simulink model "torque_controller"  (R2019a)
settings: Solver=VariableStepAuto  StartTime=0.0  StopTime=10.0  RelTol=1e-3
undefined symbols (not defined in the file): Kd, Ki, Kp
libraries: simulink x3
settings Model: Creator=Greg  LastModifiedBy=erino

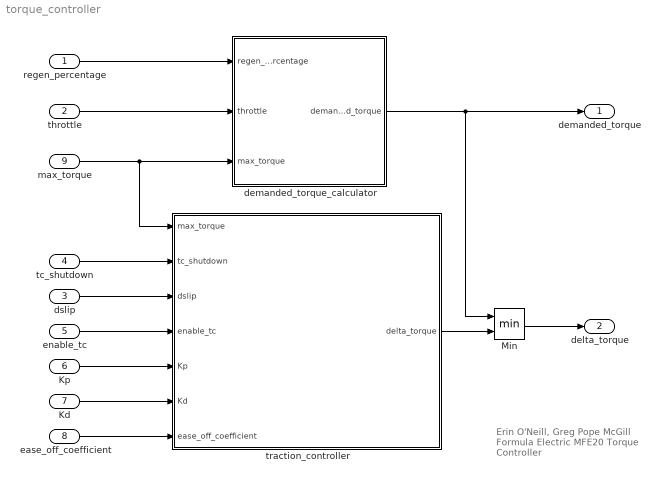
== system torque_controller ==
  note: Erin O'Neill, Greg Pope
      | McGill Formula Electric
      |
      | MFE20 Torque
      | Controller
  regen_percentage : Inport
  throttle : Inport  Port=2
  dslip : Inport  Port=3
  tc_shutdown : Inport  Port=4
  enable_tc : Inport  Port=5
  Kp : Inport  Port=6
  Kd : Inport  Port=7
  ease_off_coefficient : Inport  Port=8
  max_torque : Inport  Port=9
  Min : MinMax  Inputs=2
  demanded_torque_calculator : Subsystem
  traction_controller : Subsystem
  demanded_torque : Outport
  delta_torque : Outport  Port=2
  wires:
  Kp/1 -> traction_controller/5(Kp)
  regen_percentage/1 -> demanded_torque_calculator/1(regen_percentage)
  enable_tc/1 -> traction_controller/4(enable_tc)
  Min/1 -> delta_torque/1
  Kd/1 -> traction_controller/6(Kd)
  ease_off_coefficient/1 -> traction_controller/7(ease_off_coefficient)
  tc_shutdown/1 -> traction_controller/2(tc_shutdown)
  demanded_torque_calculator/1(demanded_torque) -> demanded_torque/1, Min/1
  dslip/1 -> traction_controller/3(dslip)
  traction_controller/1(delta_torque) -> Min/2
  throttle/1 -> demanded_torque_calculator/2(throttle)
  max_torque/1 -> traction_controller/1(max_torque), demanded_torque_calculator/3(max_torque)

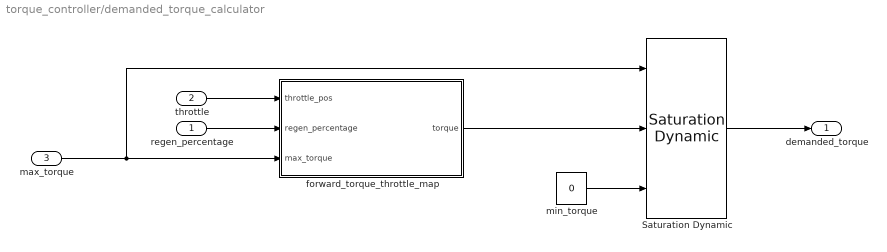
== system torque_controller/demanded_torque_calculator ==
  regen_percentage : Inport
  throttle : Inport  Port=2
  max_torque : Inport  Port=3
  Saturation Dynamic : simulink/Discontinuities/Saturation Dynamic  OutMin=[]  OutMax=[]  OutDataTypeStr=Inherit: Same as second input  OutDataType=fixdt(1, 16)  OutScaling=2^-10  DoSatur=off
  forward_torque_throttle_map : MATLAB Function  TreatAsAtomicUnit=on
  min_torque : Constant  Value=0
  demanded_torque : Outport
  wires:
  max_torque/1 -> Saturation Dynamic/1, forward_torque_throttle_map/3(max_torque)
  forward_torque_throttle_map/1(torque) -> Saturation Dynamic/2
  Saturation Dynamic/1 -> demanded_torque/1
  throttle/1 -> forward_torque_throttle_map/1(throttle_pos)
  min_torque/1 -> Saturation Dynamic/3
  regen_percentage/1 -> forward_torque_throttle_map/2(regen_percentage)

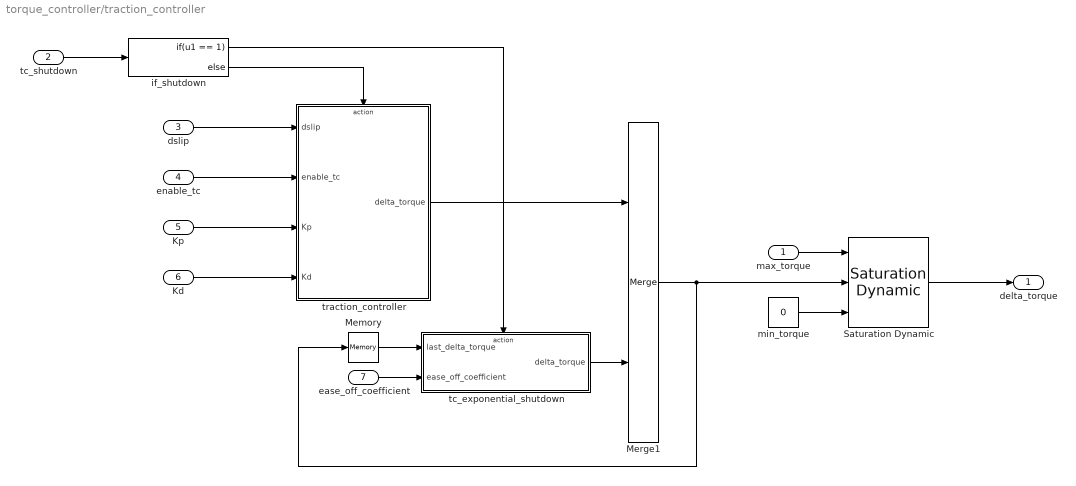
== system torque_controller/traction_controller ==
  max_torque : Inport
  tc_shutdown : Inport  Port=2
  dslip : Inport  Port=3
  enable_tc : Inport  Port=4
  Kp : Inport  Port=5
  Kd : Inport  Port=6
  ease_off_coefficient : Inport  Port=7
  Memory : Memory
  Merge1 : Merge
  Saturation Dynamic : simulink/Discontinuities/Saturation Dynamic  OutMin=[]  OutMax=[]  OutDataTypeStr=Inherit: Same as second input  OutDataType=fixdt(1, 16)  OutScaling=2^-10  DoSatur=off
  if_shutdown : If  IfExpression=u1 == 1
  min_torque : Constant  Value=0
  tc_exponential_shutdown : Subsystem  TreatAsAtomicUnit=on
  traction_controller : Subsystem  TreatAsAtomicUnit=on
  delta_torque : Outport
  wires:
  ease_off_coefficient/1 -> tc_exponential_shutdown/2(ease_off_coefficient)
  Kd/1 -> traction_controller/4(Kd)
  enable_tc/1 -> traction_controller/2(enable_tc)
  Kp/1 -> traction_controller/3(Kp)
  Merge1/1 -> Memory/1, Saturation Dynamic/2
  if_shutdown/1 -> tc_exponential_shutdown/Action
  dslip/1 -> traction_controller/1(dslip)
  Saturation Dynamic/1 -> delta_torque/1
  tc_shutdown/1 -> if_shutdown/1
  traction_controller/1(delta_torque) -> Merge1/1
  tc_exponential_shutdown/1(delta_torque) -> Merge1/2
  if_shutdown/2 -> traction_controller/Action
  max_torque/1 -> Saturation Dynamic/1
  min_torque/1 -> Saturation Dynamic/3
  Memory/1 -> tc_exponential_shutdown/1(last_delta_torque)

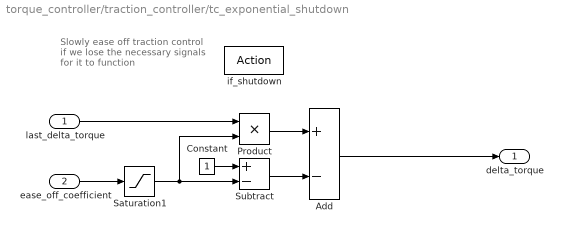
== system torque_controller/traction_controller/tc_exponential_shutdown ==
  note: Slowly ease off traction control if we lose the necessary signals for it to function
  last_delta_torque : Inport
  ease_off_coefficient : Inport  Port=2
  if_shutdown : ActionPort  ActionPortLabel=if(u1 == 1)
  Add : Sum  Inputs=+-
  Constant : Constant
  Product : Product
  Saturation1 : Saturate  UpperLimit=1  LowerLimit=0
  Subtract : Sum  Inputs=+-
  delta_torque : Outport
  wires:
  ease_off_coefficient/1 -> Saturation1/1
  last_delta_torque/1 -> Product/1
  Saturation1/1 -> Subtract/2, Product/2
  Product/1 -> Add/1
  Subtract/1 -> Add/2
  Constant/1 -> Subtract/1
  Add/1 -> delta_torque/1

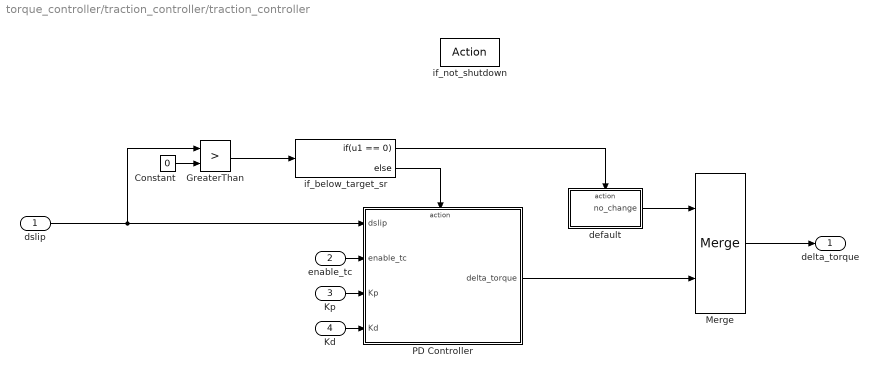
== system torque_controller/traction_controller/traction_controller ==
  dslip : Inport
  enable_tc : Inport  Port=2
  Kp : Inport  Port=3
  Kd : Inport  Port=4
  if_not_shutdown : ActionPort  ActionPortLabel=else
  Constant : Constant  Value=0
  GreaterThan : RelationalOperator  Operator=>  OutDataTypeStr=boolean  RndMeth=Simplest
  Merge : Merge
  PD Controller : Subsystem  TreatAsAtomicUnit=on
  default : Subsystem  TreatAsAtomicUnit=on
  if_below_target_sr : If  IfExpression=u1 == 0
  delta_torque : Outport
  wires:
  Merge/1 -> delta_torque/1
  default/1(no_change) -> Merge/1
  PD Controller/1(delta_torque) -> Merge/2
  dslip/1 -> PD Controller/1(dslip), GreaterThan/1
  enable_tc/1 -> PD Controller/2(enable_tc)
  Kp/1 -> PD Controller/3(Kp)
  Kd/1 -> PD Controller/4(Kd)
  GreaterThan/1 -> if_below_target_sr/1
  Constant/1 -> GreaterThan/2
  if_below_target_sr/1 -> default/Action
  if_below_target_sr/2 -> PD Controller/Action

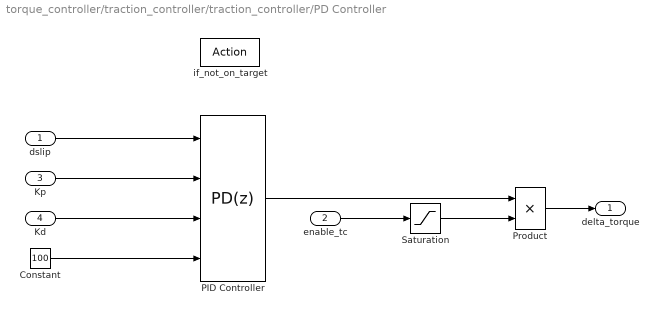
== system torque_controller/traction_controller/traction_controller/PD Controller ==
  dslip : Inport
  enable_tc : Inport  Port=2
  Kp : Inport  Port=3
  Kd : Inport  Port=4
  if_not_on_target : ActionPort  ActionPortLabel=else
  Constant : Constant  Value=100
  PID Controller : simulink/Continuous/PID Controller  Controller=PD  Form=Parallel  TimeDomain=Discrete-time  SampleTime=-1  IntegratorMethod=Forward Euler  FilterMethod=Forward Euler  ControllerParametersSource=external  P=Kp  I=Ki  D=Kd  UseFilter=on  N=100  TunerSelectOption=Transfer Function Based (PID Tuner App)  InitialConditionSource=internal  InitialConditionForIntegrator=0  InitialConditionForFilter=0  DifferentiatorICPrevScaledInput=0  ExternalReset=none  TrackingMode=off  Kt=1  LimitOutput=on  UpperSaturationLimit=240  LowerSaturationLimit=0  LinearizeAsGain=on  AntiWindupMode=none  Kb=1  POutMin=[]  POutMax=[]  IOutMin=[]  IOutMax=[]  DOutMin=[]  DOutMax=[]  NOutMin=[]  NOutMax=[]  SumOutMin=[]  SumOutMax=[]  SaturationOutMin=[]  SaturationOutMax=[]  PParamMin=[]  PParamMax=[]  IParamMin=[]  IParamMax=[]  DParamMin=[]  DParamMax=[]  NParamMin=[]  NParamMax=[]  KbParamMin=[]  KbParamMax=[]  KtParamMin=[]  KtParamMax=[]  KbOutMin=[]  KbOutMax=[]  KtOutMin=[]  KtOutMax=[]  IntegratorOutMin=[]  IntegratorOutMax=[]  FilterOutMin=[]  FilterOutMax=[]  SumI1OutMin=[]  SumI1OutMax=[]  SumI2OutMin=[]  SumI2OutMax=[]  SumI3OutMin=[]  SumI3OutMax=[]  SumI4OutMin=[]  SumI4OutMax=[]  SumDOutMin=[]  SumDOutMax=[]  DifferentiatorOutMin=[]  DifferentiatorOutMax=[]  FilterDiffOutCoefMin=[]  FilterDiffOutCoefMax=[]  ReciprocalOutMin=[]  ReciprocalOutMax=[]  SumDenOutMin=[]  SumDenOutMax=[]  SumNumOutMin=[]  SumNumOutMax=[]  DivideOutMin=[]  DivideOutMax=[]  IntegratorContinuousStateAttributes=''  IntegratorStateMustResolveToSignalObject=off  IntegratorRTWStateStorageClass=Auto  FilterContinuousStateAttributes=''  FilterStateMustResolveToSignalObject=off  FilterRTWStateStorageClass=Auto  ParallelPVariant=ExternalParameters  IdealPVariant=Disabled  IVariant=Disabled  DVariant=ExternalParameters  IntegratorVariant=Disabled  SatVariant=Enabled  AWVariant=Disabled  PCopyVariant=Disabled  TRVariant=Disabled  FdbkBlocksVariant=Forward  IdealPFdbkVariant=Disabled  SatFdbkVariant=Disabled  DerivativeFilterVariant=ForwardEulerFilter  NVariant=ExternalParameters  NCopyVariant=Disabled  FilterICVariant=InternalICsFilter  IntegratorICVariant=Disabled  ExternalResetVariant=Disabled  TRSumVariant=Passthrough  SumFdbkVariant=Disabled  SumVariant=Sum_PD
  Product : Product
  Saturation : Saturate  UpperLimit=1  LowerLimit=0  OutDataTypeStr=uint8
  delta_torque : Outport
  wires:
  dslip/1 -> PID Controller/1
  Constant/1 -> PID Controller/4
  Kd/1 -> PID Controller/3
  Product/1 -> delta_torque/1
  Saturation/1 -> Product/2
  PID Controller/1 -> Product/1
  enable_tc/1 -> Saturation/1
  Kp/1 -> PID Controller/2

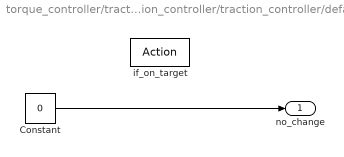
== system torque_controller/traction_controller/traction_controller/default ==
  if_on_target : ActionPort  ActionPortLabel=if(u1 == 0)
  Constant : Constant  Value=0
  no_change : Outport
  wires:
  Constant/1 -> no_change/1

== matlab function torque_controller/demanded_torque_calculator/forward_torque_throttle_map ==
  data: throttle_pos input; regen_percentage input; max_torque input; torque output
function torque = forward_torque_throttle_map(throttle_pos, regen_percentage, max_torque)

if throttle_pos <= .05 && throttle_pos >= 0 % deadzone of 5%
    torque = 0; 

elseif regen_percentage == 0
    if (throttle_pos - .05) < 0
        torque = 0; 
    else
        torque = ((throttle_pos - .05)/.95) * max_torque; % regen is off, .05 to 1 throttle is 0 to max torque
    end
    
else 
    if (throttle_pos - .1) < 0
        torque = 0; 
    else
        torque = ((throttle_pos - .1)/.9) * max_torque; % regen is on, 0.1 to 1 throttle is 0 to max torque    
    end
end

if torque < 0 
    torque = 0;
    
elseif torque > 240
    torque = 240;   
end
